simulink model "Modelo_sistema_doble_pendulo_fijo"  (R2023b)
settings: Solver=VariableStepAuto  StartTime=0.0  StopTime=10000  RelTol=1e-3
undefined symbols (not defined in the file): g, l1, l2, m1, m2
settings Model: Creator=Casa  LastModifiedBy=Casa

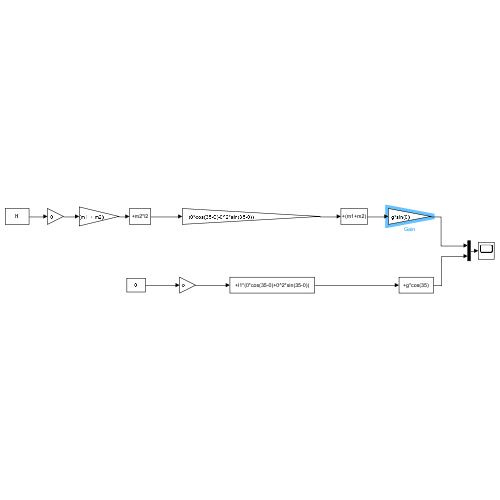
[thumbnail: Simulink's stored preview of the top-level diagram]
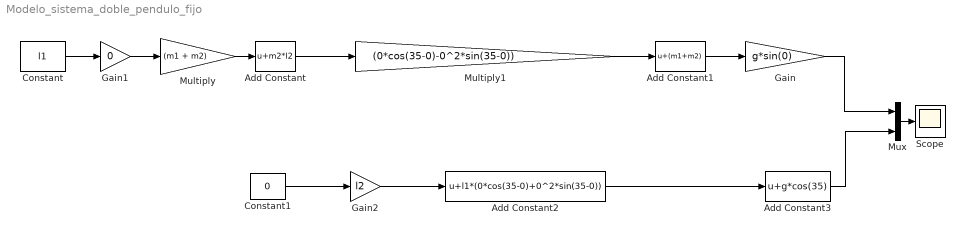
== system Modelo_sistema_doble_pendulo_fijo ==
  Add Constant : Bias  Bias=m2*l2  SaturateOnIntegerOverflow=off
  Add Constant1 : Bias  Bias=(m1+m2)  SaturateOnIntegerOverflow=off
  Add Constant2 : Bias  Bias=l1*(0*cos(35-0)+0^2*sin(35-0))  SaturateOnIntegerOverflow=off
  Add Constant3 : Bias  Bias=g*cos(35)  SaturateOnIntegerOverflow=off
  Constant : Constant  Value=l1
  Constant1 : Constant  Value=0
  Gain : Gain  Gain=g*sin(0)
  Gain1 : Gain  Gain=0
  Gain2 : Gain  Gain=l2
  Multiply : Gain  Gain=(m1 + m2)
  Multiply1 : Gain  Gain=(0*cos(35-0)-0^2*sin(35-0))
  Mux : Mux  Inputs=2
  Scope : Scope
  wires:
  Multiply/1 -> Add Constant/1
  Add Constant/1 -> Multiply1/1
  Multiply1/1 -> Add Constant1/1
  Add Constant1/1 -> Gain/1
  Add Constant2/1 -> Add Constant3/1
  Gain/1 -> Mux/1
  Add Constant3/1 -> Mux/2
  Mux/1 -> Scope/1
  Constant/1 -> Gain1/1
  Gain1/1 -> Multiply/1
  Constant1/1 -> Gain2/1
  Gain2/1 -> Add Constant2/1
